simulink model "cntrl1"  (R2013a)
settings: Solver=ode45  StartTime=0.0  StopTime=5  RelTol=1e-3
settings Model: Creator=Daniel  LastModifiedBy=Daniel

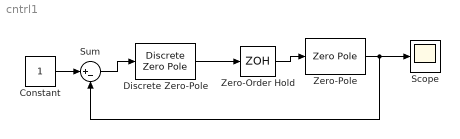
== system cntrl1 ==
  Constant : Constant
  Discrete Zero-Pole : DiscreteZeroPole  Zeros=[+.67]  Poles=[+.24]  Gain=1.31
  Scope : Scope
  Sum : Sum  Inputs=|+-
  Zero-Order Hold : ZeroOrderHold  SampleTime=.2
  Zero-Pole : ZeroPole  Zeros=[]  Poles=[0 -2]
  wires:
  Zero-Order Hold/1 -> Zero-Pole/1
  Discrete Zero-Pole/1 -> Zero-Order Hold/1
  Constant/1 -> Sum/1
  Sum/1 -> Discrete Zero-Pole/1
  Zero-Pole/1 -> Scope/1, Sum/2
